simulink model "BrickPiTest"  (R2018b)
settings: Solver=FixedStepAuto  StartTime=0.0  StopTime=inf  FixedStep=0.01  RelTol=1e-3
libraries: BrickPi x7, raspberrypilib x1
settings Model: SimulationMode=external  Creator=Isshu  LastModifiedBy=Isshu
settings SolverCC: PositivePriorityOrder=on
settings OptimizationCC: EnhancedBackFolding=on  PassReuseOutputArgsAs=Individual arguments  MaxStackSize=64  OptimizeBlockOrder=speed  DifferentSizesBufferReuse=on  OptimizationCustomize=off
settings DebuggingCC: ParameterTunabilityLossMsg=error
settings HardwareCC: ProdBitPerPointer=32  ProdBitPerSizeT=32  ProdBitPerPtrDiffT=32  ProdLargestAtomicInteger=Long  ProdLargestAtomicFloat=Double  ProdWordSize=32  ProdHWDeviceType=ARM Compatible->ARM Cortex  UseEmbeddedCoderFeatures=off  UseSimulinkCoderFeatures=off
settings ModelReferenceCC: PropagateVarSize=During execution
settings SFSimCC: MATLABDynamicMemAlloc=off
settings RTWCC: SystemTargetFile=ert.tlc  HardwareBoard=Raspberry Pi  TLCOptions="-aInlineSetEventsForThisBaseRateFcn=TLC_FALSE -aSuppressMultiTaskScheduler=TLC_FALSE  -aRateBasedStepFcn=0"  TemplateMakefile=ert_default_tmf  RTWVerbose=off  Toolchain=GNU GCC Raspberry Pi  BuildConfiguration=Faster Runs  IncludeHyperlinkInReport=on
settings CodeAppCC: ForceParamTrailComments=on  OperatorAnnotations=on  SimulinkDataObjDesc=on  SFDataObjDesc=on  MangleLength=10  InsertBlockDesc=on
settings ERTTargetCC: SupportNonInlinedSFcns=on  SupportVariableSizeSignals=on  ExtMode=on  ExtModeMexArgs='169.254.0.2' 0 17725  ERTSrcFileBannerTemplate=codertarget_code_template.cgt  ERTHdrFileBannerTemplate=codertarget_code_template.cgt  ERTDataSrcFileTemplate=codertarget_code_template.cgt  ERTDataHdrFileTemplate=codertarget_code_template.cgt

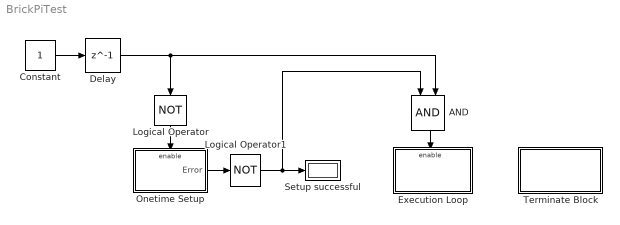
== system BrickPiTest ==
  AND : Logic  AllPortsSameDT=off  OutDataTypeStr=boolean
  Constant : Constant
  Delay : Delay  DelayLength=1
  Execution Loop : Subsystem
  Logical Operator : Logic  Operator=NOT  AllPortsSameDT=off  OutDataTypeStr=boolean
  Logical Operator1 : Logic  Operator=NOT  AllPortsSameDT=off  OutDataTypeStr=boolean
  Onetime Setup : Subsystem
  Setup successful : Display
  Terminate Block : Subsystem  TreatAsAtomicUnit=on
  wires:
  Constant/1 -> Delay/1
  Logical Operator/1 -> Onetime Setup/Enable
  Onetime Setup/1(Error) -> Logical Operator1/1
  AND/1 -> Execution Loop/Enable
  Logical Operator1/1 -> Setup successful/1, AND/1
  Delay/1 -> AND/2, Logical Operator/1

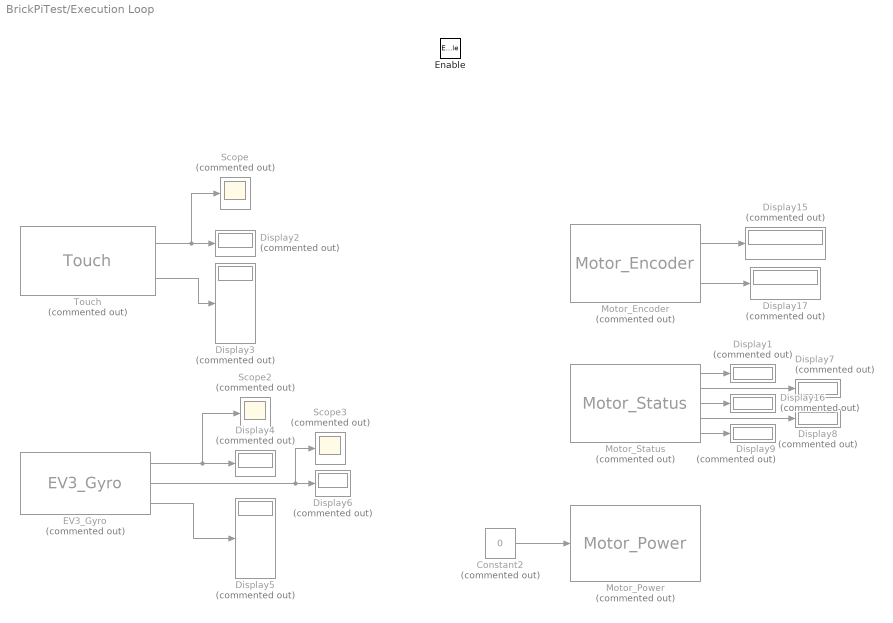
== system BrickPiTest/Execution Loop ==
  Enable : EnablePort
  Constant2 : Constant  Commented=on  Value=0  OutDataTypeStr=int8
  Display{1..9,15..17} (12 alike) : Display  Commented=on
  EV3_Gyro : BrickPi/EV3_Gyro  Commented=on  SensorPort=2  SensorType=SENSOR_TYPE_EV3_GYRO_ABS_DPS
  Motor_Encoder : BrickPi/Motor_Encoder  Commented=on  MotorPort=A  ResetMode=Reset on external signal
  Motor_Power : BrickPi/Motor_Power  Commented=on  MotorPort=A  choice=Power  Kp=0  Kd=0  Kp_DPS=0  Kd_DPS=0
      link override Power: OutDataTypeStr=int8
  Motor_Status : BrickPi/Motor_Status  Commented=on  MotorPort=A  ResetMode=Reset on external signal
  Scope : Scope  Commented=on
  Scope2 : Scope  Commented=on
  Scope3 : Scope  Commented=on
  Touch : BrickPi/Touch  Commented=on  SensorPort=1  SensorType=SENSOR_TYPE_TOUCH_EV3
  wires:
  Touch/1 -> Scope/1, Display2/1
  Touch/2 -> Display3/1
  EV3_Gyro/2 -> Scope3/1, Display6/1
  EV3_Gyro/3 -> Display5/1
  EV3_Gyro/1 -> Scope2/1, Display4/1
  Motor_Encoder/1 -> Display15/1
  Motor_Status/3 -> Display16/1
  Constant2/1 -> Motor_Power/1
  Motor_Encoder/2 -> Display17/1
  Motor_Status/1 -> Display1/1
  Motor_Status/2 -> Display7/1
  Motor_Status/4 -> Display8/1
  Motor_Status/5 -> Display9/1

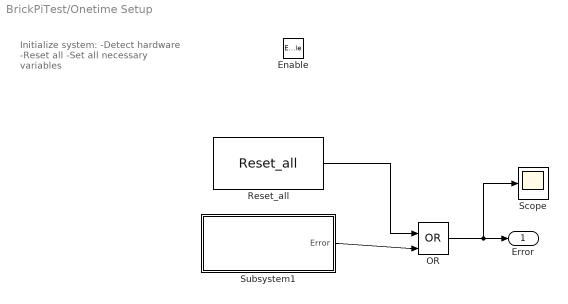
== system BrickPiTest/Onetime Setup ==
  note: Initialize system:
      |
      | -Detect hardware
      | -Reset all
      | -Set all necessary variables
  Enable : EnablePort
  OR : Logic  Operator=OR  IconShape=distinctive  AllPortsSameDT=off  OutDataTypeStr=boolean
  Reset_all : BrickPi/Reset_all  SystemSampleTime=-1
  Scope : Scope
  Subsystem1 : Subsystem  Priority=10
      mask Display:
      | disp('Get \n manufacturer')
      | port_label('output',1,'Error')
  Error : Outport  InitialOutput=[1]
  wires:
  Subsystem1/1(Error) -> OR/2
  OR/1 -> Scope/1, Error/1
  Reset_all/1 -> OR/1

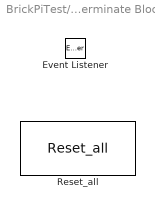
== system BrickPiTest/Terminate Block ==
  Event Listener : EventListener  DisableCoverage=on  EventType=Terminate  EventName=reset
  Reset_all : BrickPi/Reset_all  SystemSampleTime=-1

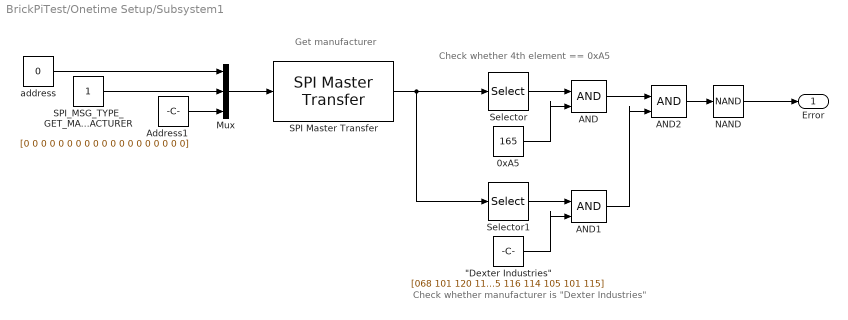
== system BrickPiTest/Onetime Setup/Subsystem1 ==
  note: Check whether 4th element == 0xA5
  note: Get manufacturer
  note: Check whether manufacturer is "Dexter Industries"
  "\"Dexter Industries\"" : Constant  Value=[068 101 120 116 101 114 032 073 110 100 117 115 116 114 105 101 115]  OutDataTypeStr=uint8
  0xA5 : Constant  Value=165  OutDataTypeStr=uint8
  AND : Logic  IconShape=distinctive  AllPortsSameDT=off  OutDataTypeStr=boolean
  AND1 : Logic  IconShape=distinctive  AllPortsSameDT=off  OutDataTypeStr=boolean
  AND2 : Logic  IconShape=distinctive  AllPortsSameDT=off  OutDataTypeStr=boolean
  Address1 : Constant  Value=[0 0 0 0 0 0 0 0 0 0 0 0 0 0 0 0 0 0 0]  OutDataTypeStr=uint8
  Mux : Mux  Inputs=3
  NAND : Logic  Operator=NAND  Inputs=1  IconShape=distinctive  AllPortsSameDT=off  OutDataTypeStr=boolean
  SPI Master Transfer : raspberrypilib/SPI Master Transfer  BoardProperty=Pi 3 Model B  SPIModule=uint32(0)  Mode=Master  BusSpeed=1000000  Pin=SPI0_CE1  FirstBitToTransfer=Most significant bit (MSB)  ClockMode=0  BlockFunction=Transfer  RegisterAddress=0  OutputDataType=int8  OutputDataLength=1
      settings: SourceProductName=Simulink Support Package for Raspberry Pi Hardware  SourceProductBaseCode=RASPPI
  SPI_MSG_TYPE_ GET_MANUFACTURER : Constant  OutDataTypeStr=uint8
  Selector : Selector  InputPortWidth=21  IndexOptions=Index vector (dialog)  Indices=[4]  OutputSizes=1
  Selector1 : Selector  InputPortWidth=21  IndexOptions=Index vector (dialog)  Indices=[5:1:21]  OutputSizes=1
  address : Constant  Value=0  OutDataTypeStr=uint8
  Error : Outport
  wires:
  SPI Master Transfer/1 -> Selector1/1, Selector/1
  Mux/1 -> SPI Master Transfer/1
  SPI_MSG_TYPE_ GET_MANUFACTURER/1 -> Mux/2
  0xA5/1 -> AND/2
  AND1/1 -> AND2/2
  Selector/1 -> AND/1
  AND/1 -> AND2/1
  "\"Dexter Industries\""/1 -> AND1/2
  address/1 -> Mux/1
  Address1/1 -> Mux/3
  Selector1/1 -> AND1/1
  AND2/1 -> NAND/1
  NAND/1 -> Error/1
